simulink model "FocParamIdentifyModel"  (R2024a)
settings: Solver=FixedStepDiscrete  StartTime=0.0  StopTime=4  FixedStep=0.00005  RelTol=1e-3
values from neighbouring files (symbols this model uses):
  Flux = 0.00084    [FocParamIDFData.mat]
  Ld = 3.62e-05    [FocParamIDFData.mat]
  Lq = 4.24e-05    [FocParamIDFData.mat]
  Pole = 10    [FocParamIDFData.mat]
  Rs = 0.113    [FocParamIDFData.mat]
  Ts = 5e-05    [FocParamIDFData.mat]
undefined symbols (not defined in the file or in its folder): DiscIntNeverNeededParam, magnitude
libraries: slpidlib x4, mcbplantlib x1, autolibpmsmexterior x1
(part 2 of 2)

== stateflow chart FocParamIdentifyModel/FocParamIDF/ParamIDF1 ==
  state Ready
    en:
    Theta = single(0.0);
    Ud_t = single(0.0);
    Rs_t = single(0.0);
    Cnt = 1;
    Tim_Total = single(0.0);
    Uq = single(0.0);
    Ud = single(0.0);
    Ld = single(0.0);
    Lq = single(0.0);
    Ld_t = single(0.0);
    Lq_t = single(0.0);
  note: Ud缓慢增加阶段
  note: 计算电阻 累加阶段
  note: 平均电阻计算阶段
  note: 等待电流稳定
  state Rs_Stage1
    en:
    du:
    Ud_t = Ud_t + single(0.0001);
    Ud = Ud_t;
  state Rs_Stage4
    en:
    Ud = single(0.0);
    Uq = single(0.0);
    Cnt = 0;
    Tim_Total = single(0.0);
  state Rs_Stage2
    en:
    du:
    Rs_t = Rs_t + (Ud_t/Id)
    Cnt = Cnt + 1;
    Tim_Total = Tim_Total + single(0.00005);
  state Rs_Stage3
    en:
    Rs = Rs_t / single(1000.0)
  state Ld_Stage5
    en:
    Ud = single(0.0);
    Uq = single(0.0);
    Cnt = 0;
    Tim_Total = single(0.0);
  state Ld_State4
    en:
    Ld = Ld_t / single(Cnt);
    Cnt = 0;
  state Ld_State1
    en:
    Ud = single(1.0);
    Uq = single(0.0);
    du:
    Tim_Total = Tim_Total + single(0.00005);
  state Ld_State2
    en:
    Ud = single(0.0);
    Uq = single(0.0);
    Ld_t = Ld_t + (single(1.0)*Tim_Total)/Id;
    Cnt = Cnt + 1;
  state Ld_State3
    en:
    Ud = single(0.0);
    Uq = single(0.0);
    Tim_Total = single(0.0);
  state Lq_Stage5
    en:
    Ud = single(0.0);
    Uq = single(0.0);
    Cnt = 0;
    Tim_Total = single(0.0);
    du:
    Tim_Total = Tim_Total + single(0.00005);
  state Lq_State4
    en:
    Lq = Lq_t / single(Cnt);
    Cnt = 0;
  state Lq_State1
    en:
    Ud = single(0.0);
    Uq = single(1.0);
    du:
    Tim_Total = Tim_Total + single(0.00005);
  state Lq_State2
    en:
    Ud = single(0.0);
    Uq = single(0.0);
    Lq_t = Lq_t + (single(1.0)*Tim_Total/Iq);
    Cnt = Cnt + 1;
  state Lq_State3
    en:
    Ud = single(0.0);
    Uq = single(0.0);
    Tim_Total = single(0.0);
  state Flux_State1
    en:
    Flux_Alpha_dot = single(0.0);
    Flux_Beta_dot = single(0.0);
    Flux_Alpha = single(0.0);
    Flux_Beta = single(0.0);
    Tim_Total = single(0.0);
    du:
    Flux_Alpha_dot = Ualpha - Rs*Ialpha;
    Flux_Beta_dot = Ubeta - Rs*Ibeta;
    Flux_Alpha = Flux_Alpha + Flux_Alpha_dot * single(0.00005);
    Flux_Beta = Flux_Beta + Flux_Beta_dot * single(0.00005);
    Flux = sqrt(Flux_Alpha*Flux_Alpha + Flux_Beta*Flux_Beta);
    if Theta < single(2*pi)
    Theta = Theta + single(0.001);
    else
    Theta = single(0.0);
    end
    Tim_Total = Tim_Total + single(0.00005);
  note: 拖动电机以we = 20rad/s的速度旋转
  state Flux_State0
    en:
    Tim_Total = single(0.0);
    Theta = 0;
    Uq = single(0.5);
    Ud = single(0.0);
    du:
    if Theta < single(2*pi)
    Theta = Theta + single(0.001);
    else
    Theta = single(0.0);
    end
    Tim_Total = Tim_Total + single(0.00005);
  state Flux_State2
    en:
    Ud = single(0.0);
    Uq = single(0.0);
    Tim_Total = single(0.0);
  note: Flux _Alpha_dot = Ualpha - Ialpha * Rs;
      | Flux_Beta_dot = Ubeta - Ibeta * Rs;
      | Flux = sqrt(Flux_Alpha² + Flux_Beta²);
  (default) -> Ready
  Rs_Stage1 -> Rs_Stage2 : [Id > 2]
  Ready -> Rs_Stage1 : [Clock > single(0.5)]
  Rs_Stage2 -> Rs_Stage3 : [Cnt > 1000]
  Rs_Stage3 -> Rs_Stage4
  Rs_Stage4 -> Ld_State1 : [Id <= single(0.001)&&Iq<= single(0.001)]
  Ld_State4 -> Ld_Stage5
  Ld_State1 -> Ld_State2 : [Tim_Total >= 0.0002]
  Ld_State3 -> Ld_State4 [order 2] : [Cnt >= 10]
  Ld_State2 -> Ld_State3
  Ld_Stage5 -> Lq_State1 : [Iq <= single(0.001) && Id <= single(0.001)]
  Ld_State3 -> Ld_State1 [order 1] : [Id < single(0.001)]
  Lq_State4 -> Lq_Stage5
  Lq_State3 -> Lq_State4 [order 2] : [Cnt >= 10]
  Lq_State2 -> Lq_State3
  Lq_State1 -> Lq_State2 : [Tim_Total >= 0.0002]
  Lq_Stage5 -> Flux_State0 : [Id <= single(0.001) && Iq <= single(0.001) && Tim_Total > single(0.5)]
  Lq_State3 -> Lq_State1 [order 1] : [Iq < single(0.001)]
  Flux_State0 -> Flux_State1 : [Tim_Total >= single(1.5)]
  Flux_State1 -> Flux_State2 : [Tim_Total > single(1.5)]
  data: Ud output single; Ud_t local single; Rs_t local single; Cnt local int16; Clock input single; Rs output single; Id input single; Uq output single; Tim_Total local single; Iq input single; Ld output single; Lq output single; Ld_t local single; Lq_t local single; Theta output single; Ealpha local single; Ebeta local single; Ubeta input single; Ualpha input single; Ialpha input single; Ibeta input single; Flux output single; Flux_Alpha_dot output single; Flux_Beta output single; Flux_Alpha output single; Flux_Beta_dot output single; Theta_Input input single
